simulink model "CBB_ccontrol_pspice_SMC"  (R2021a)
settings: Solver=VariableStepAuto  StartTime=0.0  StopTime=1  RelTol=1e-3
undefined symbols (not defined in the file): ki, kp, L, R
libraries: pspsim x1, spsSawtoothGeneratorLib x1
settings Model: Creator=omar_  LastModifiedBy=LAPONE

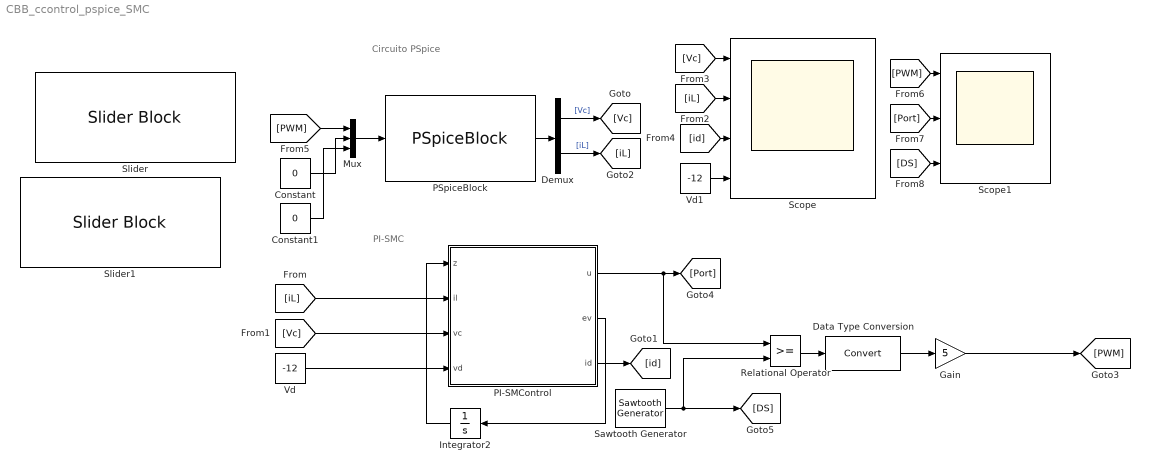
== system CBB_ccontrol_pspice_SMC ==
  note: Circuito PSpice
  note: PI-SMC
  Constant : Constant  Value=0
  Constant1 : Constant  Value=0
  Data Type Conversion : DataTypeConversion
  Demux : Demux  Outputs=2
  Gain : Gain  Gain=5
  Integrator2 : Integrator  InitialCondition=0.001
  Mux : Mux  Inputs=3
  PI-SMControl : MATLAB Function  TreatAsAtomicUnit=on
  PSpiceBlock : pspsim/PSpiceBlock  SFunctionModules=''
      settings: SourceProductName=PSpice Block
  Relational Operator : RelationalOperator  OutDataTypeStr=boolean  RndMeth=Simplest
  Sawtooth Generator : spsSawtoothGeneratorLib/Sawtooth Generator  Freq=50000  Phase=0  Ts=0
  Scope : Scope  NumInputPorts=4
  Scope1 : Scope  NumInputPorts=3
  Slider : SliderBlock  ScaleMax=3
  Slider1 : SliderBlock  ScaleMax=3
  Vd : Constant  Value=-12
  Vd1 : Constant  Value=-12
  wires:
  [DS] -> Scope1/3
  Relational Operator/1 -> Data Type Conversion/1
  [Port] -> Scope1/2
  PI-SMControl/3(id) -> [id]
  [iL] -> PI-SMControl/2(il)
  [iL] -> Scope/2
  Integrator2/1 -> PI-SMControl/1(z)
  PSpiceBlock/1 -> Demux/1
  [Vc] -> Scope/1
  Data Type Conversion/1 -> Gain/1
  Gain/1 -> [PWM]
  [Vc] -> PI-SMControl/3(vc)
  Demux/2 -> [iL]  "[iL]"
  Demux/1 -> [Vc]  "[Vc]"
  Sawtooth Generator/1 -> [DS], Relational Operator/2
  Vd/1 -> PI-SMControl/4(vd)
  [id] -> Scope/3
  PI-SMControl/2(ev) -> Integrator2/1
  [PWM] -> Scope1/1
  Mux/1 -> PSpiceBlock/1
  [PWM] -> Mux/1
  PI-SMControl/1(u) -> Relational Operator/1, [Port]
  Vd1/1 -> Scope/4
  Constant/1 -> Mux/2
  Constant1/1 -> Mux/3

== matlab function CBB_ccontrol_pspice_SMC/PI-SMControl ==
  data: E parameter; u output; ki parameter; R parameter; kp parameter; z input; il input; vc input; L parameter; vd input; ev output; id output
function [u,ev,id] = fcn(E, ki, R, kp, z,il,vc,L, vd)

il = double(il); vc = double(vc); 
ev = double(vc -vd);
id=kp*ev+ki*z;
u=(1/2)*(1-sign(il-id));
